simulink model "simSystem"  (R2024a)
settings: Solver=VariableStepAuto  StartTime=0.0  StopTime=t_sim  RelTol=1e-3
libraries: cstblocks x1, rllib x1
settings Model: Creator=lorenzo  LastModifiedBy=lorenzo

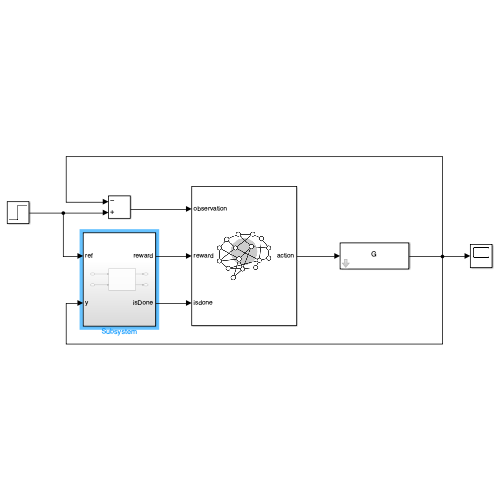
[thumbnail: Simulink's stored preview of the top-level diagram]
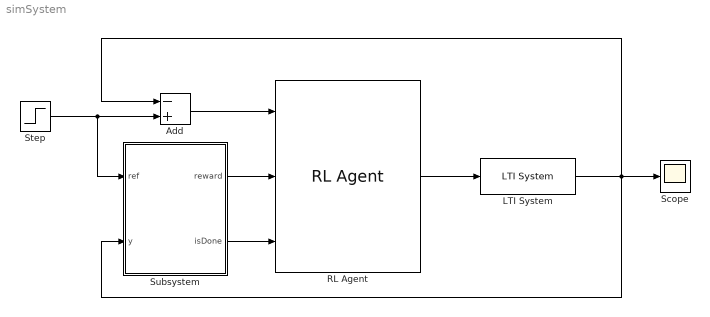
== system simSystem ==
  Add : Sum  Inputs=-+
  LTI System : cstblocks/LTI System  sys=G  IC=0  PadeOrder=0
  RL Agent : rllib/RL Agent  Agent=agent  ExternalActionAsInput=off  ProvideLastAction=off  ProvideCumRwd=off  TreatAsDirectFeedthrough=on  UseStrictObservationDataTypes=off
  Scope : Scope
  Step : Step  Time=0  SampleTime=0
  Subsystem : Subsystem
  wires:
  Add/1 -> RL Agent/1
  LTI System/1 -> Scope/1, Subsystem/2(y), Add/1
  Step/1 -> Add/2, Subsystem/1(ref)
  Subsystem/1(reward) -> RL Agent/2
  Subsystem/2(isDone) -> RL Agent/3
  RL Agent/1 -> LTI System/1

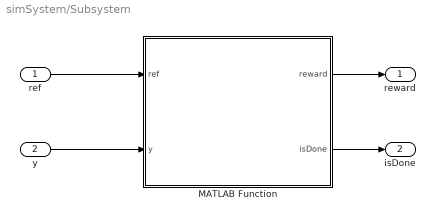
== system simSystem/Subsystem ==
  ref : Inport
  y : Inport  Port=2
  MATLAB Function : MATLAB Function  TreatAsAtomicUnit=on
  reward : Outport
  isDone : Outport  Port=2
  wires:
  ref/1 -> MATLAB Function/1(ref)
  y/1 -> MATLAB Function/2(y)
  MATLAB Function/1(reward) -> reward/1
  MATLAB Function/2(isDone) -> isDone/1

== matlab function simSystem/Subsystem/MATLAB Function ==
  data: ref input; reward output; y input; isDone output
function [reward, isDone] = fcn(ref, y)

% steady state error
error = abs(y - ref);

% overshoot
if y > ref
    overshoot = y-ref;
else
    overshoot = 0;
end


reward = -error - 3 * overshoot;
isDone = error < 0.01;
% isDone = error < 0.05 && overshoot < 0.1;
